simulink model "robust_controller"  (Simulink 7.2)
settings: Solver=FixedStepDiscrete  SolverMode=SingleTasking  StartTime=0  StopTime=inf  FixedStep=TS  RelTol=1e-3
PreLoadFcn:
  | param_nxtway_gs
values from neighbouring files (symbols this model uses):
  C_hh = [1 0]    [olp_robot_2dof.m]
undefined symbols (not defined in the file or in its folder): a_b, a_d, a_gc, a_gd, A_h, a_r, B_h, C_h, D_h, dst_thr, gp_max, k_phidot, k_sync, k_thetadot, log_count, pwm_gain, sound_dur, sound_freq, time_auto, time_start, ts1, ts2, ts3, turn_angle
libraries: ecrobot_nxt_lib x30, simulink x2
(part 2 of 2)

== system robust_controller/nxtway_app/task_ts1/Balance & Drive Control/Controller/Cal Reference/Low Path Filter ==
  note: Low Path Filter Function
      |               1-a_r
      |          ----------------
      |          1-a_r*z^(-1)
  in : Inport
  Gain2 : Gain  Orientation=left  Gain=a_r  ParameterDataType=sfix(16)  ParameterScaling=2^0  OutDataType=sfix(16)  OutScaling=2^0  OutDataTypeStr=Inherit: Same as input  ParamDataTypeStr=Inherit: Same as input
  Gain3 : Gain  Gain=1-a_r  ParameterDataType=sfix(16)  ParameterScaling=2^0  OutDataType=sfix(16)  OutScaling=2^0  OutDataTypeStr=Inherit: Same as input  ParamDataTypeStr=Inherit: Same as input
  Sum : Sum  Inputs=|++  OutDataType=sfix(16)  OutScaling=2^0  OutDataTypeStr=Inherit: Same as first input
  Unit Delay : UnitDelay  Orientation=left  SampleTime=-1
  out : Outport
  wires:
  Sum/1 -> Unit Delay/1, out/1
  Unit Delay/1 -> Gain2/1
  Gain2/1 -> Sum/2
  Gain3/1 -> Sum/1
  in/1 -> Gain3/1

== system robust_controller/nxtway_app/task_ts1/Balance & Drive Control/Controller/Cal x1/Cal gyro_offset ==
  note: Low Path Filter Function
      |               1-a_gd
      |          ----------------
      |          1-a_gd*z^(-1)
  gyro : Inport  OutDataType=sfix(16)  OutScaling=2^0
  Data Store Read1 : DataStoreRead  Priority=1  DataStoreName=gyro_offset  SampleTime=-1
  Data Store Read2 : DataStoreRead  Priority=-1  DataStoreName=gyro_offset  SampleTime=-1
  Data Store Write1 : DataStoreWrite  Priority=0  DataStoreName=gyro_offset  SampleTime=-1
  Gain1 : Gain  Gain=1-a_gd  ParameterDataType=sfix(16)  ParameterScaling=2^0  OutDataType=sfix(16)  OutScaling=2^0  OutDataTypeStr=Inherit: Same as input  ParamDataTypeStr=Inherit: Same as input
  Gain4 : Gain  Gain=a_gd  ParameterDataType=sfix(16)  ParameterScaling=2^0  OutDataType=sfix(16)  OutScaling=2^0  OutDataTypeStr=Inherit: Same as input  ParamDataTypeStr=Inherit: Same as input
  Sum : Sum  Inputs=|++  OutDataType=sfix(16)  OutScaling=2^0  OutDataTypeStr=Inherit: Same as first input
  gyro_offset : Outport  OutDataType=sfix(16)  OutScaling=2^0
  wires:
  Data Store Read1/1 -> gyro_offset/1
  Data Store Read2/1 -> Gain4/1
  Gain1/1 -> Sum/2
  Gain4/1 -> Sum/1
  Sum/1 -> Data Store Write1/1
  gyro/1 -> Gain1/1

== system robust_controller/nxtway_app/task_ts1/Balance & Drive Control/Controller/Cal x1/Discrete Derivative (backward difference) ==
  in : Inport  OutDataType=sfix(16)  OutScaling=2^0
  Gain : Gain  Gain=1/ts1  ParameterDataType=sfix(16)  ParameterScaling=2^0  OutDataType=sfix(16)  OutScaling=2^0  OutDataTypeStr=Inherit: Same as input  ParamDataTypeStr=Inherit: Same as input
  Sum : Sum  Inputs=|+-  OutDataType=sfix(16)  OutScaling=2^0  OutDataTypeStr=Inherit: Same as first input
  Unit Delay : UnitDelay  SampleTime=-1
  out : Outport  OutDataType=sfix(16)  OutScaling=2^0
  wires:
  Sum/1 -> Gain/1
  Unit Delay/1 -> Sum/2
  in/1 -> Unit Delay/1, Sum/1
  Gain/1 -> out/1

== system robust_controller/nxtway_app/task_ts1/Balance & Drive Control/Controller/Cal x1/Discrete Integrator (forward euler) ==
  in : Inport  OutDataType=sfix(16)  OutScaling=2^0
  Gain : Gain  Gain=ts1  ParameterDataType=sfix(16)  ParameterScaling=2^0  OutDataType=sfix(16)  OutScaling=2^0  OutDataTypeStr=Inherit: Same as input  ParamDataTypeStr=Inherit: Same as input
  Sum : Sum  Inputs=|++  OutDataType=sfix(16)  OutScaling=2^0  OutDataTypeStr=Inherit: Same as first input
  Unit Delay : UnitDelay  SampleTime=-1
  out : Outport  OutDataType=sfix(16)  OutScaling=2^0
  wires:
  in/1 -> Gain/1
  Sum/1 -> Unit Delay/1
  Gain/1 -> Sum/1
  Unit Delay/1 -> out/1, Sum/2

== system robust_controller/nxtway_app/task_ts1/Balance & Drive Control/Controller/Cal x1/Low Path Filter ==
  note: Low Path Filter Function
      |               1-a_d
      |          ----------------
      |          1-a_d*z^(-1)
  in : Inport
  Gain2 : Gain  Orientation=left  Gain=a_d  ParameterDataType=sfix(16)  ParameterScaling=2^0  OutDataType=sfix(16)  OutScaling=2^0  OutDataTypeStr=Inherit: Same as input  ParamDataTypeStr=Inherit: Same as input
  Gain3 : Gain  Gain=1-a_d  ParameterDataType=sfix(16)  ParameterScaling=2^0  OutDataType=sfix(16)  OutScaling=2^0  OutDataTypeStr=Inherit: Same as input  ParamDataTypeStr=Inherit: Same as input
  Sum : Sum  Inputs=|++  OutDataType=sfix(16)  OutScaling=2^0  OutDataTypeStr=Inherit: Same as first input
  Unit Delay : UnitDelay  Orientation=left  SampleTime=-1
  out : Outport
  wires:
  Sum/1 -> Unit Delay/1, out/1
  Unit Delay/1 -> Gain2/1
  Gain2/1 -> Sum/2
  Gain3/1 -> Sum/1
  in/1 -> Gain3/1

== system robust_controller/nxtway_app/task_ts1/Balance & Drive Control/Controller/Cal PWM/Cal theta_diff/Detect Flag Falling ==
  flag : Inport  OutDataType=sfix(16)  OutScaling=2^0
  Constant : Constant  Value=0  VectorParams1D=off  OutDataTypeMode=boolean  OutDataType=FIXDT  OutScaling=2^0  OutDataTypeStr=boolean  SampleTime=-1
      settings: AttributesFormatString=DataType = %<OutDataTypeStr>
  Constant1 : Constant  VectorParams1D=off  OutDataTypeMode=boolean  OutDataType=FIXDT  OutScaling=2^0  OutDataTypeStr=boolean  SampleTime=-1
      settings: AttributesFormatString=DataType = %<OutDataTypeStr>
  Logical Operator : Logic  AllPortsSameDT=off  OutDataTypeMode=boolean  OutDataTypeStr=boolean
  Relational Operator : RelationalOperator  Operator===  LogicOutDataTypeMode=boolean  OutDataTypeStr=boolean
  Relational Operator1 : RelationalOperator  Operator===  LogicOutDataTypeMode=boolean  OutDataTypeStr=boolean
  Unit Delay : UnitDelay  SampleTime=-1
  falling : Outport  OutDataType=sfix(16)  OutScaling=2^0
  wires:
  flag/1 -> Unit Delay/1, Relational Operator/1
  Constant/1 -> Relational Operator/2
  Unit Delay/1 -> Relational Operator1/1
  Constant1/1 -> Relational Operator1/2
  Relational Operator/1 -> Logical Operator/1
  Relational Operator1/1 -> Logical Operator/2
  Logical Operator/1 -> falling/1

== system robust_controller/nxtway_app/task_ts1/Balance & Drive Control/Controller/Cal PWM/Cal theta_diff/Set theta_offset ==
  theta_diff : Inport
  Enable : EnablePort
  theta_offset : Outport
  wires:
  theta_diff/1 -> theta_offset/1
